simulink library "PI_lib"  (R2020a)
settings: Solver=VariableStepAuto  StartTime=0.0  StopTime=10.0  RelTol=1e-3
settings Model: Creator=sonal  LastModifiedBy=sonal

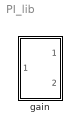
== system PI_lib ==
  gain : Subsystem  mask{A=1, B=2}
      mask Display: image('ic.jpg'); % Use "Edit Image" on toolstrip to change.

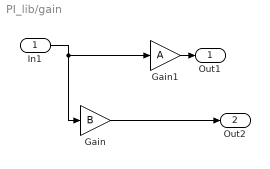
== system PI_lib/gain ==
  In1 : Inport
  Gain : Gain  Gain=B
  Gain1 : Gain  Gain=A
  Out1 : Outport
  Out2 : Outport  Port=2
  wires:
  In1/1 -> Gain1/1, Gain/1
  Gain/1 -> Out2/1
  Gain1/1 -> Out1/1
